simulink model "onefour"  (R2021a)
settings: Solver=VariableStepAuto  StartTime=0.0  StopTime=10.0  RelTol=1e-3
settings Model: Creator=Windows  LastModifiedBy=Windows

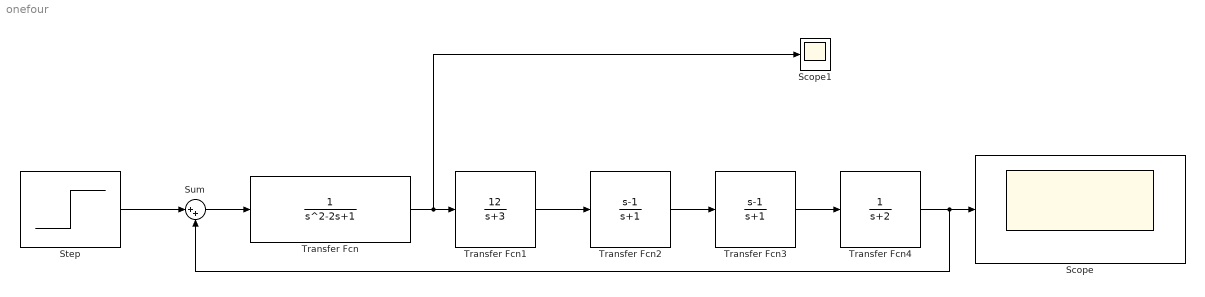
== system onefour ==
  Scope : Scope
  Scope1 : Scope
  Step : Step  SampleTime=0
  Sum : Sum  Inputs=|++
  Transfer Fcn : TransferFcn  Denominator=[1 -2 1]
  Transfer Fcn1 : TransferFcn  Numerator=[12]  Denominator=[1 3]
  Transfer Fcn2 : TransferFcn  Numerator=[1 -1]  Denominator=[1 1]
  Transfer Fcn3 : TransferFcn  Numerator=[1 -1]  Denominator=[1 1]
  Transfer Fcn4 : TransferFcn  Numerator=[1 ]  Denominator=[1 2]
  wires:
  Transfer Fcn/1 -> Scope1/1, Transfer Fcn1/1
  Transfer Fcn1/1 -> Transfer Fcn2/1
  Transfer Fcn2/1 -> Transfer Fcn3/1
  Transfer Fcn3/1 -> Transfer Fcn4/1
  Transfer Fcn4/1 -> Sum/2, Scope/1
  Step/1 -> Sum/1
  Sum/1 -> Transfer Fcn/1
